simulink model "BMS"  (R2024b)
settings: Solver=ode23tb  StartTime=0.0  StopTime=1  RelTol=1e-3  EnableMultiTasking=on
PreLoadFcn:
  | % Data of Solar Panel
  | %5000[W]/130[W]
  | % Total power generated by solar panel reaches 5[KW].
  | % each solar panel generates power 130[kW].
  | V = [0    40 80 120 160 180 200 217 240 260 280];
  | I = 5000/130*[0.68 0.675 0.67 0.665 0.660 0.655 0.640 0.6 0.48 0.28 0];
  | 
  | %subplot(211);plot(V,I);xlabel('Voltage[V]');ylabel('Current[a]')
  | %subplot(212);plot(V.*I);title('Power[W]')
  | 
  | % Sample Time[s]
  | Ts =5e-6;
  | 
  | 
  | %MPPT + PV Control
  | % PI control pamameter of Voltage control(Outer loop)
  | Kp_V = 50e-3;
  | Ki_V = 10;
  | 
  | % PI Control pamameter of Current control(Inner loop)
  | Kp_I = 25e-3;
  | Ki_I = 10;
  | 
  | % Utility Interconnection Control
  | % PI Control pamameter of Voltage control(Outer loop)
  | Kp_V2 = 0.01;
  | Ki_V2 = 25;
  | 
  | % PI control pamameter of Current control(Inner loop)
  | Kp_I2 = 0.01;
  | Ki_I2 = 25;
  | 
  | 
  | % Difference of voltege using in MPPT
  | dV = 0.5;
  | 
  | % Battery Control
  | % PI Control pamameter of Voltage control(Outer loop)
  | Kp_VB = 0.4;
  | Ki_VB = 2;
  | 
  | % PI control pamameter of Current control(Inner loop)
  | Kp_IB = 0.1;
  | Ki_IB = 0.5;
undefined symbols (not defined in the file): Acid, Ion, Lead, Lithium, sigbuilder_block
libraries: spsBreakerLib x120, spsBatteryLib x111, spsSeriesRLCBranchLib x59, spsVoltageMeasurementLib x17, spsIdealSwitchLib x15, spsMosfetLib x11, slpidlib x9, spsCurrentMeasurementLib x7, spsPWMGeneratorDCDCLib x7, spsDiodeLib x6, spsPWMGenerator2LevelLib x5, spspowerguiLib x3
(part 1 of 6)
Description:
  | Copyright 2008-2017 The MathWorks, Inc.
settings Model: SimulationMode=accelerator  Creator=MathWorks  LastModifiedBy=Jatay
settings SolverCC: ZeroCrossControl=DisableAll  ZeroCrossAlgorithm=Adaptive  AlgebraicLoopSolver=TrustRegion
settings DataIOCC: LimitDataPoints=on  SaveFormat=Array  SignalLoggingSaveFormat=ModelDataLogs  ReturnWorkspaceOutputs=off
settings OptimizationCC: ExpressionDepthLimit=2147483647  LifeSpan=inf
settings DebuggingCC: UnderspecifiedInitializationDetection=Classic  MergeDetectMultiDrivingBlocksExec=none  SolverPrmCheckMsg=warning  FcnCallInpInsideContextMsg=warning  UnconnectedInputMsg=warning  UnconnectedOutputMsg=warning  UnconnectedLineMsg=warning  AllowSymbolicDim=off  StateNameClashWarn=warning  SFUnexpectedBacktrackingDiag=warning  SFNoUnconditionalDefaultTransitionDiag=warning  SFExecutionAtInitializationDiag=none  ArithmeticOperatorsInVariantConditions=warning
settings HardwareCC: ProdBitPerPointer=32  ProdBitPerSizeT=32  ProdBitPerPtrDiffT=32  ProdLargestAtomicFloat=None  ProdIntDivRoundTo=Undefined  ProdEndianess=Unspecified  ProdWordSize=32  ProdHWDeviceType=32-bit Generic
settings ModelReferenceCC: EnableRefExpFcnMdlSchedulingChecks=on  PropagateSignalLabelsOutOfModel=off
settings SFSimCC: SimUseLocalCustomCode=off  SimParseCustomCode=off  CustomCodeUndefinedFunction=UseInterfaceOnly
settings RTWCC: RTWUseLocalCustomCode=off  GPUComputeCapability=3.5
settings CodeAppCC: StateflowObjectComments=on
settings GRTTargetCC: TargetLangStandard=C89/C90 (ANSI)  CombineOutputUpdateFcns=off  GRTInterface=on
settings ConfigComp: CovMetricSettings=dw  CovSaveCumulativeToWorkspaceVar=on  CovSaveSingleToWorkspaceVar=on  CovExternalEMLEnable=off  CovSFcnEnable=off
settings SimscapeCC: SimscapeNormalizeSystem=off

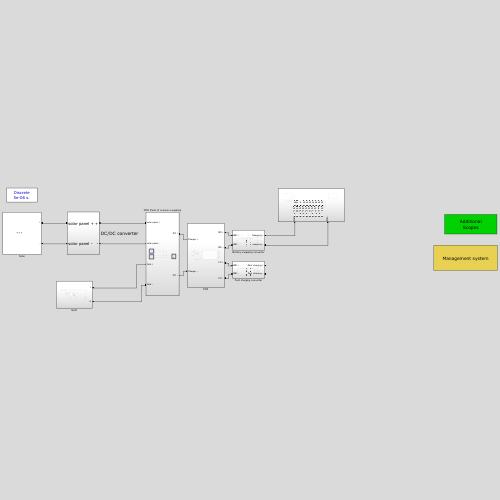
[thumbnail: Simulink's stored preview of the top-level diagram]
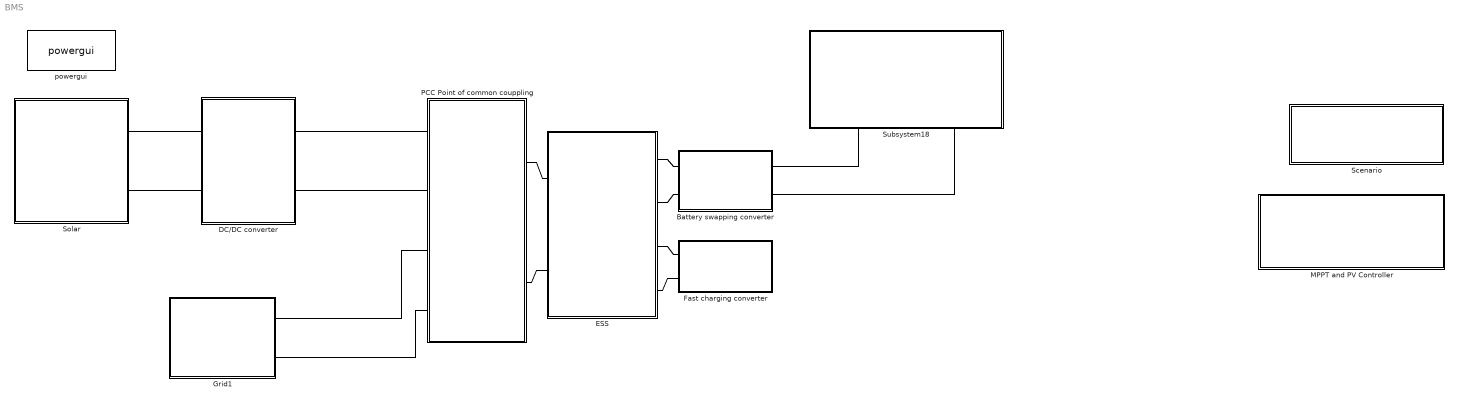
== system BMS ==
  Battery swapping converter : Subsystem
  DC/DC converter : Subsystem
  ESS : Subsystem
  Fast charging converter : Subsystem
  Grid1 : Subsystem
  MPPT and PV Controller : Subsystem
      mask Display: disp('Management system')
  PCC Point of common couppling : Subsystem
  Scenario : Subsystem
      mask Display: disp('Additional\nScopes')
  Solar : Subsystem
      mask Display: image('Solar-Power-Plant-1024x536.jpg');
  Subsystem18 : Subsystem
  powergui : spspowerguiLib/powergui  Priority=1  SimulationMode=Discrete  SampleTime=5e-6  frequency=60  Iterations=50  frequencyindice=0  Pbase=100e6  ErrMax=1e-4  UnitsV=kV  UnitsW=MW  buscounter=0  FunctionMessages=off  echomessages=off  EnableUseOfTLC=off  CurrentSourceSwitches=off  DisableSnubberDevices=off  DisableRonSwitches=off  DisableVfSwitches=off  DisplayEquations=off  AutomaticDiscreteSolvers=off  SolverType=Tustin  Interpol=off  ExternalGateDelay=off  methode=off  Ts=0  x0status=blocks  SPID=off  SwTol=0  HookPort=off  NonlinearTolerance=1e-4  nMaxIteration=100  ContinueOnMaxIteration=off  RestoreLinks=warning  ResistiveCurrentMeasurement=off  Frange=[0:2:500]  Ylog=off  Xlog=on  ShowGrid=off  save=off  variable=ZData  structure=0  ZoomFFT=off  StartTime=0.0  cycles=1  DisplayStyle=1  fundamental=60  FreqAxis=off  MaxFrequency=1000  frequencyindicesteady=1  RmsSteady=1  display=off
  connections:
  DC/DC converter/LConn2 -- Solar/RConn2
  DC/DC converter/LConn1 -- Solar/RConn1
  ESS/LConn2 -- PCC Point of common couppling/RConn2
  PCC Point of common couppling/RConn1 -- ESS/LConn1
  PCC Point of common couppling/LConn1 -- DC/DC converter/RConn1
  DC/DC converter/RConn2 -- PCC Point of common couppling/LConn2
  Grid1/RConn1 -- PCC Point of common couppling/LConn3
  Grid1/RConn2 -- PCC Point of common couppling/LConn4
  ESS/RConn1 -- Battery swapping converter/LConn1
  ESS/RConn2 -- Battery swapping converter/LConn2
  ESS/RConn3 -- Fast charging converter/LConn1
  Fast charging converter/LConn2 -- ESS/RConn4
  Subsystem18/LConn1 -- Battery swapping converter/RConn1
  Subsystem18/LConn2 -- Battery swapping converter/RConn2

== system BMS/Battery swapping converter ==
  Current Measurement : spsCurrentMeasurementLib/Current Measurement  PhasorSimulation=off  OutputType=Complex  PSBequivalent=0
  Current Measurement1 : spsCurrentMeasurementLib/Current Measurement  PhasorSimulation=off  OutputType=Complex  PSBequivalent=0
  Current Measurement2 : spsCurrentMeasurementLib/Current Measurement  PhasorSimulation=off  OutputType=Complex  PSBequivalent=0
  Diode : spsDiodeLib/Diode  Ron=0.001  Lon=0  Vf=0.8  IC=0  UseSnubber=0  Rs=500  Cs=250e-9  Measurements=off
  Mosfet : spsMosfetLib/Mosfet  Ron=0.1  Lon=0  Rd=0.01  Vfd=0  IC=0  Rs=1e5  Cs=inf  Measurements=off
  Product : Product
  Pulse Generator : DiscretePulseGenerator  PulseType=Time based  Period=10  PulseWidth=5
  Scope2 : Scope  NumInputPorts=3
  Scope3 : Scope
  Scope4 : Scope
  Series RLC Branch : spsSeriesRLCBranchLib/Series RLC Branch  LConnTagsString=__new0  RConnTagsString=__new0  BranchType=L  Resistance=1  Inductance=1e-3  SetiL0=off  InitialCurrent=0  Capacitance=1e-6  Setx0=off  InitialVoltage=0  Measurements=None
  Series RLC Branch2 : spsSeriesRLCBranchLib/Series RLC Branch  LConnTagsString=__new0  RConnTagsString=__new0  BranchType=C  Resistance=1  Inductance=1e-3  SetiL0=off  InitialCurrent=0  Capacitance=1e-6  Setx0=off  InitialVoltage=0  Measurements=None
  Voltage Measurement : spsVoltageMeasurementLib/Voltage Measurement  PhasorSimulation=off  OutputType=Complex  PSBequivalent=0
  BB + : PMIOPort  Side=Left
  BB - : PMIOPort  Port=2  Side=Left
  Swapping + : PMIOPort  Port=3  Side=Right
  swapping - : PMIOPort  Port=4  Side=Right
  wires:
  Current Measurement/1 -> Scope2/1
  Voltage Measurement/1 -> Scope4/1, Product/1
  Current Measurement1/1 -> Scope2/3, Product/2
  Product/1 -> Scope3/1
  Current Measurement2/1 -> Scope2/2
  Pulse Generator/1 -> Mosfet/1
  connections:
  Series RLC Branch2/RConn1 -- BB -/RConn1 -- Series RLC Branch/RConn1 -- swapping -/RConn1 -- Voltage Measurement/LConn2
  Diode/LConn1 -- Current Measurement1/LConn1 -- Series RLC Branch2/LConn1
  BB +/RConn1 -- Current Measurement/LConn1
  Current Measurement1/RConn1 -- Swapping +/RConn1 -- Voltage Measurement/LConn1
  Mosfet/RConn1 -- Diode/RConn1 -- Current Measurement2/LConn1
  Current Measurement/RConn1 -- Mosfet/LConn1
  Current Measurement2/RConn1 -- Series RLC Branch/LConn1

== system BMS/DC//DC converter ==
  Bidirectional DC/DC Converter : Subsystem
  DC - DC Converter : Subsystem
  DC bus : Subsystem
  Voltage Measurement2 : spsVoltageMeasurementLib/Voltage Measurement  PhasorSimulation=off  OutputType=Complex  PSBequivalent=0
  solar panel + : PMIOPort  Side=Left
  solar panel - : PMIOPort  Port=2  Side=Left
  + : PMIOPort  Port=3  Side=Right
  - : PMIOPort  Port=4  Side=Right
  tag scope: solar_controller=global
  wires:
  Voltage Measurement2/1 -> [solar_controller]
  connections:
  DC - DC Converter/RConn1 -- DC bus/LConn1
  solar panel +/RConn1 -- DC - DC Converter/LConn1 -- Voltage Measurement2/LConn1
  DC - DC Converter/LConn2 -- Voltage Measurement2/LConn2 -- solar panel -/RConn1
  DC - DC Converter/RConn2 -- DC bus/LConn2
  Bidirectional DC/DC Converter/LConn1 -- DC bus/RConn1
  Bidirectional DC/DC Converter/LConn2 -- DC bus/RConn2
  -/RConn1 -- Bidirectional DC/DC Converter/RConn2
  Bidirectional DC/DC Converter/RConn1 -- +/RConn1

== system BMS/ESS ==
  Display : Display
  Ideal Switch : spsIdealSwitchLib/Ideal Switch  Ron=0.001  Lon=0  IC=0  Rs=1e5  Cs=inf  Measurements=off
  Subsystem : Subsystem
  Charger + : PMIOPort  Side=Left
  Charger - : PMIOPort  Port=2  Side=Left
  BS + : PMIOPort  Port=3  Side=Right
  BS - : PMIOPort  Port=4  Side=Right
  FC + : PMIOPort  Port=5  Side=Right
  FC - : PMIOPort  Port=6  Side=Right
  wires:
  [ss] -> Display/1, Ideal Switch/1
  connections:
  Ideal Switch/LConn1 -- Charger +/RConn1
  Charger -/RConn1 -- Subsystem/LConn2
  Ideal Switch/RConn1 -- Subsystem/LConn1
  FC -/RConn1 -- BS -/RConn1 -- Subsystem/RConn2
  Subsystem/RConn1 -- BS +/RConn1 -- FC +/RConn1

== system BMS/Fast charging converter ==
  Current Measurement : spsCurrentMeasurementLib/Current Measurement  PhasorSimulation=off  OutputType=Complex  PSBequivalent=0
  Current Measurement1 : spsCurrentMeasurementLib/Current Measurement  PhasorSimulation=off  OutputType=Complex  PSBequivalent=0
  Current Measurement2 : spsCurrentMeasurementLib/Current Measurement  PhasorSimulation=off  OutputType=Complex  PSBequivalent=0
  Diode : spsDiodeLib/Diode  Ron=0.001  Lon=0  Vf=0.8  IC=0  UseSnubber=0  Rs=500  Cs=250e-9  Measurements=off
  Mosfet : spsMosfetLib/Mosfet  Ron=0.1  Lon=0  Rd=0.01  Vfd=0  IC=0  Rs=1e5  Cs=inf  Measurements=off
  Product : Product
  Pulse Generator : DiscretePulseGenerator  PulseType=Time based  Period=10  PulseWidth=5
  Scope2 : Scope  NumInputPorts=3
  Scope3 : Scope
  Scope4 : Scope
  Series RLC Branch : spsSeriesRLCBranchLib/Series RLC Branch  LConnTagsString=__new0  RConnTagsString=__new0  BranchType=L  Resistance=1  Inductance=1e-3  SetiL0=off  InitialCurrent=0  Capacitance=1e-6  Setx0=off  InitialVoltage=0  Measurements=None
  Series RLC Branch2 : spsSeriesRLCBranchLib/Series RLC Branch  LConnTagsString=__new0  RConnTagsString=__new0  BranchType=C  Resistance=1  Inductance=1e-3  SetiL0=off  InitialCurrent=0  Capacitance=1e-6  Setx0=off  InitialVoltage=0  Measurements=None
  Voltage Measurement : spsVoltageMeasurementLib/Voltage Measurement  PhasorSimulation=off  OutputType=Complex  PSBequivalent=0
  BB + : PMIOPort  Side=Left
  BB - : PMIOPort  Port=2  Side=Left
  Fast charging + : PMIOPort  Port=3  Side=Right
  Fast charging - : PMIOPort  Port=4  Side=Right
  wires:
  Current Measurement/1 -> Scope2/1
  Voltage Measurement/1 -> Scope4/1, Product/1
  Current Measurement1/1 -> Scope2/3, Product/2
  Product/1 -> Scope3/1
  Current Measurement2/1 -> Scope2/2
  Pulse Generator/1 -> Mosfet/1
  connections:
  Voltage Measurement/LConn2 -- Fast charging -/RConn1 -- Series RLC Branch2/RConn1 -- Series RLC Branch/RConn1 -- BB -/RConn1
  Diode/LConn1 -- Current Measurement1/LConn1 -- Series RLC Branch2/LConn1
  BB +/RConn1 -- Current Measurement/LConn1
  Current Measurement1/RConn1 -- Voltage Measurement/LConn1 -- Fast charging +/RConn1
  Mosfet/RConn1 -- Diode/RConn1 -- Current Measurement2/LConn1
  Current Measurement/RConn1 -- Mosfet/LConn1
  Current Measurement2/RConn1 -- Series RLC Branch/LConn1

== system BMS/Grid1 ==
  Display : Display
  Grid : spsThreePhaseSourceLib/Three-Phase Source  InternalConnection=Yg  VoltagePhases=off  Voltage=380  PhaseAngle=0  Voltage_phases=[25e3 25e3 25e3]/sqrt(3)  PhaseAngles_phases=[0 -120 +120]  Frequency=50  NonIdealSource=on  SpecifyImpedance=on  Resistance=0.8929  Inductance=16.58e-3  ShortCircuitLevel=100e6  BaseVoltage=380  XRratio=7  BusType=swing  Pref=10e3  Qref=0  Prefabc=[10e3, 10e3, 10e3]  Qrefabc=[0, 0, 0]  Qmin=-inf  Qmax=inf
  LOAD1 : spsThreePhaseSeriesRLCLoadLib/Three-Phase Series RLC Load  LConnTagsString=A|B|C  Configuration=Y (grounded)  NominalVoltage=380  Vabc=[1e3 1e3 1e3]  Vabcp=[1e3 1e3 1e3]  NominalFrequency=50  UnbalancedPower=off  ActivePower=1e3  InductivePower=0  CapacitivePower=0  Pabc=[10e3 9e3 11e3]  QLabc=[100 90 110]  QCabc=[100 90 110]  Pabcp=[10e3 9e3 11e3]  QLabcp=[100 90 110]  QCabcp=[100 90 110]  Measurements=None  LoadType=constant Z
  Measurement : spsThreePhaseVIMeasurementLib/Three-Phase V-I Measurement  VoltageMeasurement=phase-to-phase  SetLabelV=on  LabelV=Vabc_grid  Vpu=off  VpuLL=off  CurrentMeasurement=yes  SetLabelI=on  LabelI=Iabc_grid  Ipu=off  Pbase=100e6  Vbase=500e3  OutputType=Complex  PhasorSimulation=off  PSBequivalent=0
  Mux : Mux  Inputs=2
  Repeating Sequence Stair : simulink/Sources/Repeating Sequence Stair  OutValues=[0 0 1 1 0].'  tsamp=0.1  OutMin=[]  OutMax=[]  OutDataTypeStr=double  OutputDataTypeScalingMode=double  OutDataType=fixdt(0,8)  ConRadixGroup=Best Precision: Vector-wise  OutScaling=2^-12
  Scope : Scope
  Scope1 : Scope
  Scope2 : Scope  NumInputPorts=2
  V2G & G2V results : Scope  NumInputPorts=3
  Voltage Measurement : spsVoltageMeasurementLib/Voltage Measurement  PhasorSimulation=off  OutputType=Complex  PSBequivalent=0
  Wall charger Connection Box : Subsystem
  + : PMIOPort  Side=Right
  +1 : PMIOPort  Port=2  Side=Right
  tag scope: Control=global
  wires:
  [Control] -> Wall charger Connection Box/1(Control)
  Mux/1 -> V2G & G2V results/3
  [Vabc_grid] -> V2G & G2V results/1
  [Vabc_inv] -> V2G & G2V results/2
  Repeating Sequence Stair/1 -> [Control], Scope1/1
  [Vabc_inv] -> Mux/2
  [Iabc_out] -> Scope2/2
  [Iabc_inv] -> Scope/1
  [Vabc_out] -> Scope2/1
  Voltage Measurement/1 -> Display/1
  [Vabc_grid] -> Mux/1
  connections:
  Wall charger Connection Box/RConn2 -- Voltage Measurement/LConn2 -- +1/RConn1
  Grid/RConn1 -- Measurement/LConn1
  Grid/RConn3 -- Measurement/LConn3
  Wall charger Connection Box/RConn1 -- Voltage Measurement/LConn1 -- +/RConn1
  Grid/RConn2 -- Measurement/LConn2
  LOAD1/LConn3 -- Wall charger Connection Box/LConn3 -- Measurement/RConn3
  Measurement/RConn2 -- Wall charger Connection Box/LConn2 -- LOAD1/LConn2
  Measurement/RConn1 -- Wall charger Connection Box/LConn1 -- LOAD1/LConn1

== system BMS/MPPT and PV Controller ==
  Battery controller : Subsystem
  Inverter controller : Subsystem
  MMPT Controller : Subsystem
  Solar controller : Subsystem
  Swapping battery controller : Subsystem

== system BMS/PCC Point of common couppling ==
  note: ESS
  note: Grid
  note: Solar
  DC + : PMIOPort  Side=Right
  solar panel + : PMIOPort  Port=2  Side=Left
  solar panel - : PMIOPort  Port=3  Side=Left
  DC - : PMIOPort  Port=4  Side=Right
  Grid + : PMIOPort  Port=5  Side=Left
  Grid - : PMIOPort  Port=6  Side=Left
  connections:
  DC +/RConn1 -- solar panel +/RConn1 -- Grid +/RConn1
  solar panel -/RConn1 -- Grid -/RConn1 -- DC -/RConn1

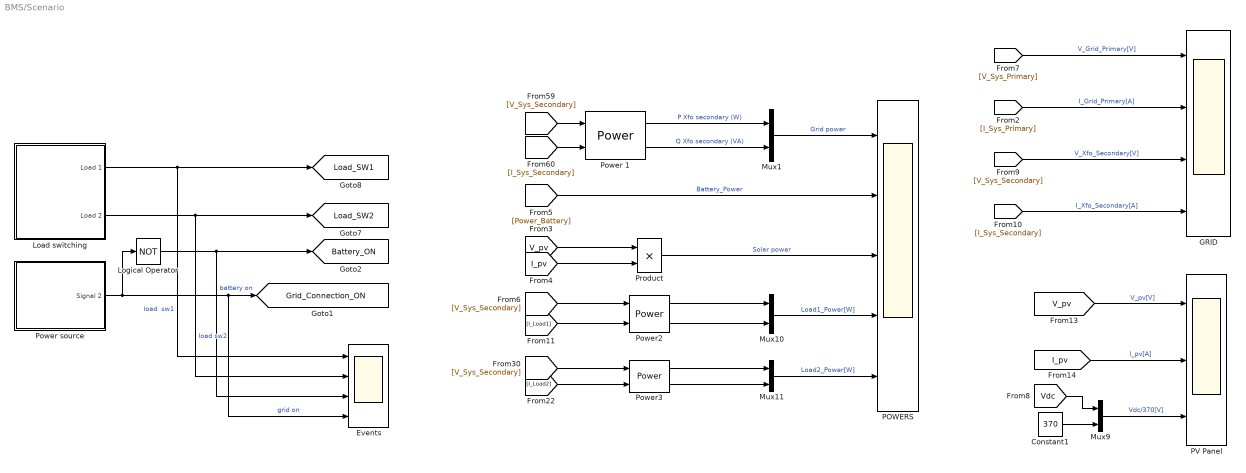
== system BMS/Scenario ==
  Constant1 : Constant  Value=370
  Events : Scope  NumInputPorts=4
  GRID : Scope  NumInputPorts=4
  Load switching : Subsystem  Tag=STV Subsys  LoadFcn=sigbuilder_block('load');  StartFcn=sigbuilder_block('start');  StopFcn=sigbuilder_block('stop');  ClipboardFcn=sigbuilder_block('clipboard');  mask(Sigbuilder block){tuvar=[0:10]}
      mask help: Simulink:masks:SigbuilderBlock_MD
      mask init:
      | if ~strcmp(get_param(bdroot(gcbh),'SimulationStatus'),'stopped') tuvar = sigbuilder_block('maskInit'); end
      settings: CopyFcn=sigbuilder_block('copy');  DeleteFcn=sigbuilder_block('delete');  ModelCloseFcn=sigbuilder_block('modelClose');  PreSaveFcn=sigbuilder_block('preSave');  PauseFcn=sigbuilder_block('pause');  ContinueFcn=sigbuilder_block('continue');  NameChangeFcn=sigbuilder_block('namechange');  OpenFcn=sigbuilder_block('open',[57 105.75 1180.5 663.75 ]);  CloseFcn=sigbuilder_block('close');
      mask Display: plot(0, 0, 100, 100,[2, 2, 32, 32, 2], [68, 8, 8, 68, 68],[32, 2], [38, 38], [32, 19, 2],[53, 60, 44], [32, 17, 17, 2],[16, 16, 31, 31]);txt = getActiveGroup(gcbh);text(2, 100, txt,'verticalAlignment', 'top');
  Logical Operator : Logic  Operator=NOT  AllPortsSameDT=off  OutDataTypeStr=boolean
  Mux{1,9..11} (4 alike) : Mux  Inputs=2
  POWERS : Scope  NumInputPorts=5
  PV Panel : Scope  NumInputPorts=3
  Power 1 : spsPowerLib/Power  Freq=60  Vinit=[1, 0]  Iinit=[1, 0]  Ts=0
  Power source : Subsystem  Tag=STV Subsys  LoadFcn=sigbuilder_block('load');  StartFcn=sigbuilder_block('start');  StopFcn=sigbuilder_block('stop');  ClipboardFcn=sigbuilder_block('clipboard');  mask(Sigbuilder block){tuvar=[0:10]}
      mask help: Simulink:masks:SigbuilderBlock_MD
      mask init:
      | if ~strcmp(get_param(bdroot(gcbh),'SimulationStatus'),'stopped') tuvar = sigbuilder_block('maskInit'); end
      settings: CopyFcn=sigbuilder_block('copy');  DeleteFcn=sigbuilder_block('delete');  ModelCloseFcn=sigbuilder_block('modelClose');  PreSaveFcn=sigbuilder_block('preSave');  PauseFcn=sigbuilder_block('pause');  ContinueFcn=sigbuilder_block('continue');  NameChangeFcn=sigbuilder_block('namechange');  OpenFcn=sigbuilder_block('open',[436.966 199.241 549.931 400.345 ]);  CloseFcn=sigbuilder_block('close');
      mask Display: plot(0, 0, 100, 100,[2, 2, 32, 32, 2], [68, 8, 8, 68, 68],[32, 2], [38, 38], [32, 19, 2],[53, 60, 44], [32, 17, 17, 2],[16, 16, 31, 31]);txt = getActiveGroup(gcbh);text(2, 100, txt,'verticalAlignment', 'top');
  Power2 : spsPowerLib/Power  Freq=60  Vinit=[1, 0]  Iinit=[1, 0]  Ts=0
  Power3 : spsPowerLib/Power  Freq=60  Vinit=[1, 0]  Iinit=[1, 0]  Ts=0
  Product : Product  RndMeth=Zero
  tag scope: Battery_ON=global, Grid_Connection_ON=global, Load_SW1=global, Load_SW2=global
  wires:
  Load switching/2(Load 2) -> [Load_SW2], Events/2  "load sw2"
  Logical Operator/1 -> Events/3, [Battery_ON]  "battery on"
  Power source/1(Signal 2) -> Events/4, [Grid_Connection_ON], Logical Operator/1  "grid on"
  Load switching/1(Load 1) -> [Load_SW1], Events/1  "load  sw1"
  [Vdc] -> Mux9/1
  Constant1/1 -> Mux9/2
  Mux9/1 -> PV Panel/3  "Vdc/370[V]"
  [V_Sys_Primary] -> GRID/1  "V_Grid_Primary[V]"
  [I_Sys_Primary] -> GRID/2  "I_Grid_Primary[A]"
  [V_Sys_Secondary] -> GRID/3  "V_Xfo_Secondary[V]"
  [I_Sys_Secondary] -> GRID/4  "I_Xfo_Secondary[A]"
  [V_pv] -> PV Panel/1  "V_pv[V]"
  [I_pv] -> PV Panel/2  "I_pv[A]"
  [V_pv] -> Product/1
  [I_pv] -> Product/2
  Product/1 -> POWERS/3  "Solar power"
  [Power_Battery] -> POWERS/2  "Battery_Power"
  [V_Sys_Secondary] -> Power 1/1
  [I_Sys_Secondary] -> Power 1/2
  [V_Sys_Secondary] -> Power2/1
  [I_Load1] -> Power2/2
  Mux10/1 -> POWERS/4  "Load1_Power[W]"
  [V_Sys_Secondary] -> Power3/1
  [I_Load2] -> Power3/2
  Mux11/1 -> POWERS/5  "Load2_Power[W]"
  Power2/1 -> Mux10/1
  Power2/2 -> Mux10/2
  Power3/1 -> Mux11/1
  Power3/2 -> Mux11/2
  Mux1/1 -> POWERS/1  "Grid power"
  Power 1/1 -> Mux1/1  "P Xfo secondary (W)"
  Power 1/2 -> Mux1/2  "Q Xfo secondary (VA)"

== system BMS/Solar ==
  note: 30 KW PV MPPT System
  "      " : ManualSwitch  CurrentSetting=0
  "      1" : ManualSwitch  CurrentSetting=0
  30 kW PV Array : spsPVArrayLib/PV Array  Npar=15  Nser=10  PlotType=array @ 1000 W/m2 & specified temperatures  S_vec="[ 1000  500  100 ]"  Temp_C_vec="[ 45 25  ]"  ModuleName=User-defined  PlotWhenSelected=off  Pm=213.15  Ncell=60  Voc=48  Isc=7.84  Vm=29  Im=7.35  beta_Voc_pc=-0.36099  alpha_Isc_pc=0.102  beta_Voc=-0.17328  alpha_Isc=0.0079968  IL=8.2285  I0=2.9956e-10  nI=1.2955  Rsh=7353.5939  Rs=2.0228  RobustModel=off  RobustCellTemperature=25  BAL=on  Tc=1e-6  Tfilter=5e-5
  Constant : Constant  Value=1000
  Constant3 : Constant  Value=25
  Current Measurement1 : spsCurrentMeasurementLib/Current Measurement  PhasorSimulation=off  OutputType=Complex  PSBequivalent=0
  Demux : Demux  Outputs=5
  Digital Clock : DigitalClock  SampleTime=0.001
  Diode : spsDiodeLib/Diode  Ron=0.5  Lon=0  Vf=0.7  IC=0  UseSnubber=0  Rs=1e5  Cs=250e-9  Measurements=off
  Diode1 : spsDiodeLib/Diode  Ron=0.5  Lon=0  Vf=0.7  IC=0  UseSnubber=0  Rs=1e5  Cs=250e-9  Measurements=off
  "Irradiance " : Subsystem  Tag=STV Subsys  LoadFcn=sigbuilder_block('load');  StartFcn=sigbuilder_block('start');  StopFcn=sigbuilder_block('stop');  ClipboardFcn=sigbuilder_block('clipboard');  mask(Sigbuilder block){tuvar=[0:10]}
      mask help: Sigbuilder GUI
      mask init:
      | if ~strcmp(get_param(bdroot(gcbh),'SimulationStatus'),'stopped') tuvar = sigbuilder_block('maskInit'); end
      settings: CopyFcn=sigbuilder_block('copy');  DeleteFcn=sigbuilder_block('delete');  ModelCloseFcn=sigbuilder_block('modelClose');  PreSaveFcn=sigbuilder_block('preSave');  PauseFcn=sigbuilder_block('pause')  ContinueFcn=sigbuilder_block('continue')  NameChangeFcn=sigbuilder_block('namechange');  OpenFcn=sigbuilder_block('open',[5.4 30 1141.2 507.6 ]);  CloseFcn=sigbuilder_block('close');
      mask Display: plot(0, 0, 100, 100,[2, 2, 32, 32, 2], [68, 8, 8, 68, 68],[32, 2], [38, 38], [32, 19, 2],[53, 60, 44], [32, 17, 17, 2],[16, 16, 31, 31]);txt = getActiveGroup(gcbh);text(2, 100, txt,'verticalAlignment', 'top');
  MPPT : Subsystem
  MPPT Power : Product
  Mosfet : spsMosfetLib/Mosfet  Ron=0.1  Lon=0  Rd=0.01  Vfd=0.7  IC=0  Rs=1e5  Cs=inf  Measurements=off
  Mux1 : Mux  Inputs=2
  PV Power : Product
  PWM Generator (DC-DC) : spsPWMGeneratorDCDCLib/PWM Generator (DC-DC)  Fsw=1500  Ts=0
  Scope : Scope  NumInputPorts=5
  Scope{1..3,5} (4 alike) : Scope
  Scope6 : Scope  NumInputPorts=3
  Scope7 : Scope  NumInputPorts=3
  Series RLC Branch : spsSeriesRLCBranchLib/Series RLC Branch  LConnTagsString=__new0  RConnTagsString=__new0  BranchType=L  Resistance=0.001  Inductance=0.4e-1  SetiL0=off  InitialCurrent=0  Capacitance=1e-6  Setx0=off  InitialVoltage=0  Measurements=None
  Series RLC Branch1 : spsSeriesRLCBranchLib/Series RLC Branch  LConnTagsString=__new0  RConnTagsString=__new0  BranchType=R  Resistance=11  Inductance=0.1  SetiL0=off  InitialCurrent=0  Capacitance=100e-6  Setx0=off  InitialVoltage=0  Measurements=None
  Series RLC Branch2 : spsSeriesRLCBranchLib/Series RLC Branch  LConnTagsString=__new0  RConnTagsString=__new0  BranchType=C  Resistance=6  Inductance=0.1  SetiL0=off  InitialCurrent=0  Capacitance=700e-5  Setx0=off  InitialVoltage=0  Measurements=None
  Series RLC Branch3 : spsSeriesRLCBranchLib/Series RLC Branch  LConnTagsString=__new0  RConnTagsString=__new0  BranchType=C  Resistance=6  Inductance=0.1  SetiL0=off  InitialCurrent=0  Capacitance=1000e-5  Setx0=off  InitialVoltage=0  Measurements=None
  Voltage Measurement : spsVoltageMeasurementLib/Voltage Measurement  PhasorSimulation=off  OutputType=Complex  PSBequivalent=0
  Voltage Measurement1 : spsVoltageMeasurementLib/Voltage Measurement  PhasorSimulation=off  OutputType=Complex  PSBequivalent=0
  + : PMIOPort  Side=Right
  - : PMIOPort  Port=2  Side=Right
  tag scope: I_pv=global, V_pv=global
  wires:
  Voltage Measurement/1 -> MPPT Power/2, Mux1/2, Scope7/2  "DC -DC Boost Converter Voltage"
  PWM Generator (DC-DC)/1 -> Mosfet/1
  Demux/1 -> Scope7/1, PV Power/1, [V_pv], MPPT/1("V _ PV "), Scope/1  "PV Voltage"
  Mux1/1 -> Scope1/1
  MPPT Power/1 -> Scope6/2, Scope2/1  "PO"
  Demux/2 -> PV Power/2, [I_pv], MPPT/2(I_PV), Scope/2
  Current Measurement1/1 -> MPPT Power/1, Mux1/1
  Voltage Measurement1/1 -> Scope3/1
  Demux/3 -> Scope/3
  Demux/4 -> Scope6/3, Scope7/3, Scope/4  "Irradiance"
  Digital Clock/1 -> MPPT/3(clock)
  MPPT/1(Duty) -> PWM Generator (DC-DC)/1
  PV Power/1 -> Scope6/1, Scope5/1
  Demux/5 -> Scope/5
  "Irradiance "/2(Temp) -> "      1"/1
  Constant3/1 -> "      1"/2
  "Irradiance "/1(Ir) -> "      "/2
  Constant/1 -> "      "/1
  "      "/1 -> 30 kW PV Array/1
  "      1"/1 -> 30 kW PV Array/2
  30 kW PV Array/1 -> Demux/1
  connections:
  Voltage Measurement/LConn2 -- 30 kW PV Array/RConn2 -- Diode1/LConn1 -- Series RLC Branch2/RConn1 -- Mosfet/RConn1 -- Voltage Measurement1/LConn2 -- Series RLC Branch3/RConn1 -- Series RLC Branch1/RConn1 -- -/RConn1
  Current Measurement1/RConn1 -- Series RLC Branch1/LConn1 -- Voltage Measurement/LConn1 -- +/RConn1
  Diode/RConn1 -- Series RLC Branch3/LConn1 -- Current Measurement1/LConn1
  Voltage Measurement1/LConn1 -- Series RLC Branch/RConn1 -- Mosfet/LConn1 -- Diode/LConn1
  Series RLC Branch2/LConn1 -- 30 kW PV Array/RConn1 -- Diode1/RConn1 -- Series RLC Branch/LConn1

== system BMS/Subsystem18 ==
  note: B1
  note: B2
  note: B3
  note: B4
  note: B5
  note: B6
  note: B13
  note: B14
  note: B15
  note: B16
  note: B17
  note: B18
  note: B19
  note: B20
  note: B21
  note: B22
  note: B7
  note: B8
  note: B9
  note: B10
  note: B11
  note: B12
  note: B23
  note: B24
  note: B25
  note: B26
  note: B27
  note: B28
  note: B29
  note: B30
  . : Subsystem
  Display : Display
  Subsystem : Subsystem
  Subsystem10 : Subsystem
  Subsystem11 : Subsystem
  Subsystem12 : Subsystem
  Subsystem13 : Subsystem
  Subsystem14 : Subsystem
  Subsystem15 : Subsystem
  Subsystem16 : Subsystem
  Subsystem17 : Subsystem
  Subsystem18 : Subsystem
  Subsystem19 : Subsystem
  Subsystem2 : Subsystem
  Subsystem20 : Subsystem
  Subsystem21 : Subsystem
  Subsystem22 : Subsystem
  Subsystem23 : Subsystem
  Subsystem24 : Subsystem
  Subsystem25 : Subsystem
  Subsystem26 : Subsystem
  Subsystem27 : Subsystem
  Subsystem28 : Subsystem
  Subsystem29 : Subsystem
  Subsystem3 : Subsystem
  Subsystem4 : Subsystem
  Subsystem5 : Subsystem
  Subsystem6 : Subsystem
  Subsystem7 : Subsystem
  Subsystem8 : Subsystem
  Subsystem9 : Subsystem
  Swapping battery controller : Subsystem
  Voltage Measurement : spsVoltageMeasurementLib/Voltage Measurement  PhasorSimulation=off  OutputType=Complex  PSBequivalent=0
  powergui : spspowerguiLib/powergui  Priority=1  SimulationMode=Continuous  SampleTime=50e-6  frequency=60  Iterations=50  frequencyindice=0  Pbase=100e6  ErrMax=1e-4  UnitsV=kV  UnitsW=MW  buscounter=0  FunctionMessages=off  echomessages=off  EnableUseOfTLC=off  CurrentSourceSwitches=off  DisableSnubberDevices=off  DisableRonSwitches=off  DisableVfSwitches=off  DisplayEquations=off  AutomaticDiscreteSolvers=off  SolverType=Tustin/Backward Euler (TBE)  Interpol=off  ExternalGateDelay=off  methode=off  Ts=100  x0status=blocks  SPID=on  SwTol=0  HookPort=off  NonlinearTolerance=1e-4  nMaxIteration=100  ContinueOnMaxIteration=off  RestoreLinks=warning  ResistiveCurrentMeasurement=off  Frange=[0:2:500]  Ylog=off  Xlog=on  ShowGrid=off  save=off  variable=ZData  structure=0  ZoomFFT=off  StartTime=0.0  cycles=1  DisplayStyle=1  fundamental=60  FreqAxis=off  MaxFrequency=1000  frequencyindicesteady=1  RmsSteady=1  display=off
  BB + : PMIOPort  Side=Left
  BB - : PMIOPort  Port=2  Side=Left
  wires:
  Voltage Measurement/1 -> Display/1
  connections:
  ./RConn2 -- Subsystem21/RConn2 -- Subsystem19/RConn2 -- Subsystem9/RConn2 -- Subsystem8/RConn2 -- Subsystem11/RConn2 -- Subsystem12/RConn2 -- Subsystem10/RConn2 -- Subsystem6/RConn2 -- Subsystem13/RConn2 -- Subsystem14/RConn2 -- Subsystem7/RConn2 -- Subsystem17/RConn2 -- Subsystem28/RConn2 -- Subsystem27/RConn2 -- Subsystem16/RConn2 -- Subsystem26/RConn2 -- Subsystem23/RConn2 -- Subsystem22/RConn2 -- Subsystem25/RConn2 -- Subsystem24/RConn2 -- Subsystem18/RConn2 -- Subsystem20/RConn2 -- Subsystem2/RConn2 -- Subsystem/RConn2 -- Subsystem3/RConn2 -- Subsystem4/RConn2 -- Voltage Measurement/LConn2 -- BB -/RConn1
  Subsystem10/RConn1 -- Subsystem7/RConn1 -- Subsystem17/RConn1 -- Subsystem29/RConn1 -- Subsystem29/RConn2 -- Subsystem28/RConn1 -- Subsystem27/RConn1 -- Subsystem16/RConn1 -- Subsystem26/RConn1 -- Subsystem25/RConn1 -- Subsystem22/RConn1 -- Subsystem23/RConn1 -- Subsystem24/RConn1 -- Subsystem15/RConn1 -- Subsystem15/RConn2 -- Subsystem14/RConn1 -- Subsystem13/RConn1 -- Subsystem6/RConn1 -- Subsystem12/RConn1 -- Subsystem11/RConn1 -- Subsystem8/RConn1 -- Subsystem20/RConn1 -- Voltage Measurement/LConn1 -- BB +/RConn1 -- ./RConn1 -- Subsystem5/RConn1 -- Subsystem5/RConn2 -- Subsystem4/RConn1 -- Subsystem3/RConn1 -- Subsystem/RConn1 -- Subsystem2/RConn1 -- Subsystem21/RConn1 -- Subsystem18/RConn1 -- Subsystem19/RConn1 -- Subsystem9/RConn1

== system BMS/DC//DC converter/Bidirectional DC//DC Converter ==
  C : spsSeriesRLCBranchLib/Series RLC Branch  LConnTagsString=__new0  RConnTagsString=__new0  BranchType=C  Resistance=1  Inductance=1e-3  SetiL0=off  InitialCurrent=0  Capacitance=1000e-6  Setx0=on  InitialVoltage=200  Measurements=None
  IGBT1 : spsIGBTDiodeLib/IGBT//Diode  Ron=1e-3  Rs=1e5  Cs=inf  Measurements=off
  IGBT2 : spsIGBTDiodeLib/IGBT//Diode  Ron=1e-3  Rs=1e5  Cs=inf  Measurements=off
  L : spsSeriesRLCBranchLib/Series RLC Branch  LConnTagsString=__new0  RConnTagsString=__new0  BranchType=L  Resistance=1  Inductance=470e-6*5  SetiL0=off  InitialCurrent=0  Capacitance=1000e-6  Setx0=off  InitialVoltage=0  Measurements=None
  Switch{1..4} (4 alike) : spsIdealSwitchLib/Ideal Switch  Ron=0.001  Lon=0  IC=0  Rs=1e6  Cs=inf  Measurements=off
  Batt + : PMIOPort  Side=Left
  Batt - : PMIOPort  Port=2  Side=Left
  + : PMIOPort  Port=3  Side=Right
  - : PMIOPort  Port=4  Side=Right
  wires:
  [G2_B] -> IGBT2/1
  [G1_B] -> IGBT1/1
  [Battery_ON] -> Switch3/1
  [Battery_ON] -> Switch1/1, Switch2/1
  [Battery_ON] -> Switch4/1
  connections:
  IGBT2/LConn1 -- L/RConn1 -- IGBT1/RConn1
  L/LConn1 -- Switch3/LConn1 -- C/LConn1
  Switch3/RConn1 -- +/RConn1
  Switch4/RConn1 -- -/RConn1
  Switch1/RConn1 -- IGBT1/LConn1
  Switch4/LConn1 -- C/RConn1 -- IGBT2/RConn1 -- Switch2/RConn1
  Batt -/RConn1 -- Switch2/LConn1
  Switch1/LConn1 -- Batt +/RConn1

== system BMS/DC//DC converter/DC - DC Converter ==
  C : spsSeriesRLCBranchLib/Series RLC Branch  LConnTagsString=__new0  RConnTagsString=__new0  BranchType=C  Resistance=0.01  Inductance=1e-3  SetiL0=off  InitialCurrent=0  Capacitance=1000e-6  Setx0=on  InitialVoltage=200  Measurements=None
  Diode : spsDiodeLib/Diode  Ron=0.001  Lon=0  Vf=1.1  IC=0  UseSnubber=off  Rs=500  Cs=250e-9  Measurements=off
  Diode2 : spsDiodeLib/Diode  Ron=0.001  Lon=0  Vf=0.7  IC=0  UseSnubber=off  Rs=500  Cs=250e-9  Measurements=off
  IGBT : spsIGBTLib/IGBT  Ron=0.001  Lon=0  Vf=1.1  Tf=1e-6  Tt=2e-6  IC=0  Rs=1e5  Cs=inf  Measurements=off
  RL : spsSeriesRLCBranchLib/Series RLC Branch  LConnTagsString=__new0  RConnTagsString=__new0  BranchType=RL  Resistance=0.05  Inductance=470e-6  SetiL0=off  InitialCurrent=0  Capacitance=1e-6  Setx0=off  InitialVoltage=0  Measurements=None
  DC + : PMIOPort  Side=Right
  solar panel + : PMIOPort  Port=2  Side=Left
  solar panel - : PMIOPort  Port=3  Side=Left
  DC - : PMIOPort  Port=4  Side=Right
  wires:
  [Pulse_PV] -> IGBT/1
  connections:
  Diode/RConn1 -- DC +/RConn1
  Diode2/RConn1 -- C/LConn1 -- RL/LConn1
  Diode/LConn1 -- RL/RConn1 -- IGBT/LConn1
  solar panel +/RConn1 -- Diode2/LConn1
  C/RConn1 -- solar panel -/RConn1 -- DC -/RConn1 -- IGBT/RConn1

== system BMS/DC//DC converter/DC bus ==
  1 ohm 2000uH : spsSeriesRLCBranchLib/Series RLC Branch  LConnTagsString=__new0  RConnTagsString=__new0  BranchType=RC  Resistance=1  Inductance=0  SetiL0=off  InitialCurrent=0  Capacitance=2000e-6  Setx0=on  InitialVoltage=370  Measurements=None
  RL + : spsSeriesRLCBranchLib/Series RLC Branch  LConnTagsString=__new0  RConnTagsString=__new0  BranchType=RL  Resistance=0.05  Inductance=470e-6  SetiL0=off  InitialCurrent=0  Capacitance=1e-6  Setx0=off  InitialVoltage=0  Measurements=None
  RL - : spsSeriesRLCBranchLib/Series RLC Branch  LConnTagsString=__new0  RConnTagsString=__new0  BranchType=RL  Resistance=0.05  Inductance=470e-6  SetiL0=off  InitialCurrent=0  Capacitance=1e-6  Setx0=off  InitialVoltage=0  Measurements=None
  Transfer Fcn : TransferFcn  Denominator=[1e-4 1]
  V : spsVoltageMeasurementLib/Voltage Measurement  PhasorSimulation=off  OutputType=Complex  PSBequivalent=0
  left + : PMIOPort  Side=Left
  left - : PMIOPort  Port=2  Side=Left
  right + : PMIOPort  Port=3  Side=Right
  right - : PMIOPort  Port=4  Side=Right
  tag scope: Vdc=global
  wires:
  V/1 -> Transfer Fcn/1
  Transfer Fcn/1 -> [Vdc]
  connections:
  RL +/RConn1 -- 1 ohm 2000uH/LConn1 -- right +/RConn1 -- V/LConn1
  RL -/RConn1 -- 1 ohm 2000uH/RConn1 -- right -/RConn1 -- V/LConn2
  left +/RConn1 -- RL +/LConn1
  left -/RConn1 -- RL -/LConn1

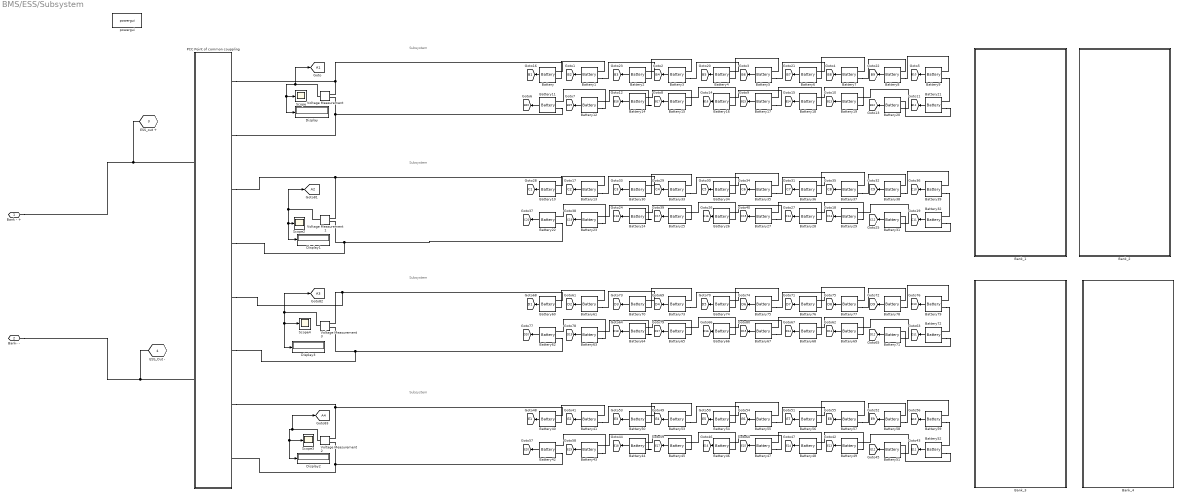
== system BMS/ESS/Subsystem ==
  note: Subsystem
  note: Subsystem
  note: Subsystem
  note: Subsystem
  Bank_1 : Subsystem
  Bank_2 : Subsystem
  Bank_3 : Subsystem
  Bank_4 : Subsystem
  Battery{,1..79} (80 alike) : spsBatteryLib/Battery  BatType=Lead-Acid  NomV=12  NomQ=100  SOC=80  Batt_Tr=10  PresetModel=on  MaxQ=104.1667  MinV=9  FullV=13.0658  Dis_rate=20  R=0.0012  Normal_OP=31.0278  expZone="[12.2171     0.333333]"
  Display{,1..3} (4 alike) : Display
  PCC Point of common couppling : Subsystem
  Scope{,2..4} (4 alike) : Scope
  Voltage Measurement{,1..3} (4 alike) : spsVoltageMeasurementLib/Voltage Measurement  PhasorSimulation=off  OutputType=Complex  PSBequivalent=0
  powergui : spspowerguiLib/powergui  Priority=1  SimulationMode=Continuous  SampleTime=50e-6  frequency=60  Iterations=50  frequencyindice=0  Pbase=100e6  ErrMax=1e-4  UnitsV=kV  UnitsW=MW  buscounter=0  FunctionMessages=off  echomessages=off  EnableUseOfTLC=off  CurrentSourceSwitches=off  DisableSnubberDevices=off  DisableRonSwitches=off  DisableVfSwitches=off  DisplayEquations=off  AutomaticDiscreteSolvers=off  SolverType=Tustin/Backward Euler (TBE)  Interpol=off  ExternalGateDelay=off  methode=off  Ts=100  x0status=blocks  SPID=on  SwTol=0  HookPort=off  NonlinearTolerance=1e-4  nMaxIteration=100  ContinueOnMaxIteration=off  RestoreLinks=warning  ResistiveCurrentMeasurement=off  Frange=[0:2:500]  Ylog=off  Xlog=on  ShowGrid=off  save=off  variable=ZData  structure=0  ZoomFFT=off  StartTime=0.0  cycles=1  DisplayStyle=1  fundamental=60  FreqAxis=off  MaxFrequency=1000  frequencyindicesteady=1  RmsSteady=1  display=off
  Bank - + : PMIOPort  Side=Left
  Bank- - : PMIOPort  Port=2  Side=Left
  ESS_out + : PMIOPort  Port=3  Side=Right
  ESS_Out - : PMIOPort  Port=4  Side=Right
  tag scope: A1=global, A2=global, A3=global, A4=global, B10=global, B11=global, B12=global, B13=global, B14=global, B15=global, B16=global, B17=global, B18=global, B19=global, B1=global, B20=global, B2=global, B3=global, B4=global, B5=global, B6=global, B7=global, B8=global, B9=global, C10=global, C11=global, C12=global, C13=global, C14=global, C15=global, C16=global, C17=global, C18=global, C19=global, C1=global, C20=global, C2=global, C3=global, C4=global, C5=global, C6=global, C7=global, C8=global, C9=global, D10=global, D11=global, D12=global, D13=global, D14=global, D15=global, D16=global, D17=global, D18=global, D19=global, D1=global, D20=global, D2=global, D3=global, D4=global, D5=global, D6=global, D7=global, D8=global, D9=global, E10=global, E11=global, E12=global, E13=global, E14=global, E15=global, E16=global, E17=global, E18=global, E19=global, E1=global, E20=global, E2=global, E3=global, E4=global, E5=global, E6=global, E7=global, E8=global, E9=global
  wires:
  Voltage Measurement/1 -> [A1], Scope/1, Display/1
  Battery1/1 -> [B2]
  Battery5/1 -> [B6]
  Battery25/1 -> [C17]
  Battery53/1 -> [E4]
  Battery20/1 -> [B12]
  Battery34/1 -> [C5]
  Battery28/1 -> [C14]
  Battery4/1 -> [B5]
  Battery45/1 -> [E17]
  Battery56/1 -> [E7]
  Voltage Measurement2/1 -> [A4], Scope3/1, Display2/1
  Battery16/1 -> [B16]
  Battery2/1 -> [B3]
  Battery18/1 -> [B14]
  Battery14/1 -> [B18]
  Voltage Measurement3/1 -> [A3], Display3/1, Scope4/1
  Battery8/1 -> [B9]
  Battery6/1 -> [B7]
  Battery17/1 -> [B15]
  Battery79/1 -> [D10]
  Battery65/1 -> [D17]
  Battery24/1 -> [C18]
  Battery9/1 -> [B10]
  Battery12/1 -> [B19]
  Battery61/1 -> [D2]
  Battery15/1 -> [B17]
  Battery21/1 -> [B11]
  Battery57/1 -> [E8]
  Battery11/1 -> [B20]
  Battery10/1 -> [C1]
  Battery64/1 -> [D18]
  Battery19/1 -> [B13]
  Battery73/1 -> [D4]
  Battery3/1 -> [B4]
  Battery41/1 -> [E2]
  Battery7/1 -> [B8]
  Battery49/1 -> [E13]
  Battery55/1 -> [E6]
  Battery66/1 -> [D16]
  Battery44/1 -> [E18]
  Battery58/1 -> [E9]
  Battery74/1 -> [D5]
  Battery42/1 -> [E20]
  Battery27/1 -> [C15]
  Battery43/1 -> [E19]
  Battery54/1 -> [E5]
  Battery48/1 -> [E14]
  Battery47/1 -> [E15]
  Battery13/1 -> [C2]
  Battery52/1 -> [E11]
  Battery59/1 -> [E10]
  Battery51/1 -> [E12]
  Battery/1 -> [B1]
  Battery50/1 -> [E3]
  Battery40/1 -> [E1]
  Battery46/1 -> [E16]
  Voltage Measurement1/1 -> [A2], Display1/1, Scope2/1
  Battery63/1 -> [D19]
  Battery38/1 -> [C9]
  Battery22/1 -> [C20]
  Battery39/1 -> [C10]
  Battery71/1 -> [D12]
  Battery32/1 -> [C11]
  Battery37/1 -> [C8]
  Battery33/1 -> [C4]
  Battery60/1 -> [D1]
  Battery35/1 -> [C6]
  Battery23/1 -> [C19]
  Battery29/1 -> [C13]
  Battery69/1 -> [D13]
  Battery31/1 -> [C12]
  Battery36/1 -> [C7]
  Battery30/1 -> [C3]
  Battery26/1 -> [C16]
  Battery70/1 -> [D3]
  Battery68/1 -> [D14]
  Battery75/1 -> [D6]
  Battery72/1 -> [D11]
  Battery62/1 -> [D20]
  Battery77/1 -> [D8]
  Battery67/1 -> [D15]
  Battery76/1 -> [D7]
  Battery78/1 -> [D9]
  connections:
  Battery61/LConn2 -- Battery70/LConn1
  Battery7/LConn2 -- Battery8/LConn1
  Battery54/LConn2 -- Battery55/LConn1
  Battery63/LConn2 -- Battery62/LConn1
  Voltage Measurement3/LConn2 -- Battery62/LConn2 -- PCC Point of common couppling/LConn6
  Battery20/LConn2 -- Battery19/LConn1
  Battery9/LConn2 -- Battery21/LConn1
  Battery56/LConn2 -- Battery57/LConn1
  Battery43/LConn2 -- Battery42/LConn1
  Battery/LConn1 -- PCC Point of common couppling/LConn1 -- Voltage Measurement/LConn1
  Battery40/LConn1 -- Voltage Measurement2/LConn1 -- PCC Point of common couppling/LConn7
  PCC Point of common couppling/LConn2 -- Battery11/LConn2 -- Voltage Measurement/LConn2
  Voltage Measurement3/LConn1 -- Battery60/LConn1 -- PCC Point of common couppling/LConn5
  Battery68/LConn2 -- Battery67/LConn1
  Battery2/LConn2 -- Battery3/LConn1
  Battery13/LConn2 -- Battery30/LConn1
  Battery39/LConn2 -- Battery32/LConn1
  Battery15/LConn2 -- Battery14/LConn1
  Battery16/LConn2 -- Battery15/LConn1
  Battery42/LConn2 -- Voltage Measurement2/LConn2 -- PCC Point of common couppling/LConn8
  Battery52/LConn2 -- Battery51/LConn1
  Battery14/LConn2 -- Battery12/LConn1
  Battery21/LConn2 -- Battery20/LConn1
  Battery6/LConn2 -- Battery7/LConn1
  Battery12/LConn2 -- Battery11/LConn1
  Battery18/LConn2 -- Battery17/LConn1
  Battery17/LConn2 -- Battery16/LConn1
  Battery3/LConn2 -- Battery4/LConn1
  Battery19/LConn2 -- Battery18/LConn1
  Battery53/LConn2 -- Battery54/LConn1
  Battery8/LConn2 -- Battery9/LConn1
  Battery26/LConn2 -- Battery25/LConn1
  Battery1/LConn2 -- Battery2/LConn1
  Battery60/LConn2 -- Battery61/LConn1
  Battery69/LConn2 -- Battery68/LConn1
  Battery50/LConn2 -- Battery53/LConn1
  Battery4/LConn2 -- Battery5/LConn1
  Battery5/LConn2 -- Battery6/LConn1
  Battery/LConn2 -- Battery1/LConn1
  Battery41/LConn2 -- Battery50/LConn1
  Battery49/LConn2 -- Battery48/LConn1
  Battery58/LConn2 -- Battery59/LConn1
  Battery48/LConn2 -- Battery47/LConn1
  Battery57/LConn2 -- Battery58/LConn1
  Battery55/LConn2 -- Battery56/LConn1
  Battery45/LConn2 -- Battery44/LConn1
  Battery40/LConn2 -- Battery41/LConn1
  Battery46/LConn2 -- Battery45/LConn1
  Battery59/LConn2 -- Battery52/LConn1
  Battery44/LConn2 -- Battery43/LConn1
  Battery76/LConn2 -- Battery77/LConn1
  Battery51/LConn2 -- Battery49/LConn1
  Battery47/LConn2 -- Battery46/LConn1
  Battery23/LConn2 -- Battery22/LConn1
  Battery10/LConn1 -- Voltage Measurement1/LConn1 -- PCC Point of common couppling/LConn3
  Battery25/LConn2 -- Battery24/LConn1
  Battery70/LConn2 -- Battery73/LConn1
  Battery10/LConn2 -- Battery13/LConn1
  Battery72/LConn2 -- Battery71/LConn1
  Battery28/LConn2 -- Battery27/LConn1
  Battery73/LConn2 -- Battery74/LConn1
  Battery74/LConn2 -- Battery75/LConn1
  Battery29/LConn2 -- Battery28/LConn1
  Battery33/LConn2 -- Battery34/LConn1
  Battery32/LConn2 -- Battery31/LConn1
  Voltage Measurement1/LConn2 -- Battery22/LConn2 -- PCC Point of common couppling/LConn4
  Battery30/LConn2 -- Battery33/LConn1
  Battery34/LConn2 -- Battery35/LConn1
  Battery38/LConn2 -- Battery39/LConn1
  Battery35/LConn2 -- Battery36/LConn1
  Battery24/LConn2 -- Battery23/LConn1
  Battery31/LConn2 -- Battery29/LConn1
  Battery36/LConn2 -- Battery37/LConn1
  Battery66/LConn2 -- Battery65/LConn1
  Battery37/LConn2 -- Battery38/LConn1
  Battery79/LConn2 -- Battery72/LConn1
  Battery27/LConn2 -- Battery26/LConn1
  Battery67/LConn2 -- Battery66/LConn1
  Battery77/LConn2 -- Battery78/LConn1
  Battery65/LConn2 -- Battery64/LConn1
  Battery78/LConn2 -- Battery79/LConn1
  Battery71/LConn2 -- Battery69/LConn1
  Battery64/LConn2 -- Battery63/LConn1
  Battery75/LConn2 -- Battery76/LConn1
  Bank - +/RConn1 -- ESS_out +/RConn1 -- PCC Point of common couppling/RConn1
  Bank- -/RConn1 -- ESS_Out -/RConn1 -- PCC Point of common couppling/RConn2

== system BMS/Grid1/Wall charger Connection Box ==
  Control : Inport
  Battery Switching Control : Subsystem
      settings: PortSchema="{\"entries\":[{\"content\":{\"sides\":[{\"content\":{\"connectorIds\":[\"LConn1\",\"LConn2\",\"LConn3\",\"LConn4\"]},\"type\":\"ConnectorPlacement.EquallySpacedRectSide\",\"uuid\":\"597ce45f-d2da-489f-9702-c83ae9b1152a\"},{\"content\":{\"connectorIds\":[\"In1\",\"RConn1\",\"RConn2\"],\"side\":\"RIGHT\"},\"type\":\"ConnectorPlacement.EquallySpacedRectSide\",\"uuid\":\"90ab1945-2787-45d6-b647-1c8eb49fe34d\"},{\"content\":{\"connectorIds\":[],\"side\":\"TOP\"},\"type\":\"ConnectorPlacement.EquallySpacedRectSide\",\"uuid\":\"5514c8fd-a1bb-4ed7-b1c0-08bce6a0e9e5\"}]},\"type\":\"ConnectorPlacement.EquallySpacedConnector\",\"uuid\":\"b6d566cb-31ba-40ab-ae9a-003997b713cb\"}],\"packageUris\":[\"http://schema.mathworks.com/mf0/Connector/R2020b\"],\"version\":\"1.0\"}"
  Buck-Boost Converter : Subsystem
  Connection Control : Subsystem
      settings: PortSchema="{\"entries\":[{\"content\":{\"sides\":[{\"content\":{\"connectorIds\":[\"LConn1\",\"LConn2\",\"LConn3\"]},\"type\":\"ConnectorPlacement.EquallySpacedRectSide\",\"uuid\":\"27ebf5cb-61b2-431e-8de2-c9344a0dfca5\"},{\"content\":{\"connectorIds\":[\"In1\",\"RConn1\",\"RConn2\",\"RConn3\",\"RConn4\",\"RConn5\",\"RConn6\"],\"side\":\"RIGHT\"},\"type\":\"ConnectorPlacement.EquallySpacedRectSide\",\"uuid\":\"2438100a-e43b-42f7-afa1-1af449516139\"},{\"content\":{\"connectorIds\":[],\"side\":\"TOP\"},\"type\":\"ConnectorPlacement.EquallySpacedRectSide\",\"uuid\":\"dcfa608d-f6dc-42e3-abf8-45a08af22825\"}]},\"type\":\"ConnectorPlacement.EquallySpacedConnector\",\"uuid\":\"5f0f36e8-f735-4489-a6f2-39fec655b509\"}],\"packageUris\":[\"http://schema.mathworks.com/mf0/Connector/R2020b\"],\"version\":\"1.0\"}"
  DC-AC / AC-DC Converter : Subsystem
  DC-DC converter with battery controller : Subsystem
  Grid_R : PMIOPort  Side=Left
  Grid_Y : PMIOPort  Port=2  Side=Left
  Grid_B : PMIOPort  Port=3  Side=Left
  Vehicle+ : PMIOPort  Port=4  Side=Right
  Vehicle- : PMIOPort  Port=5  Side=Right
  wires:
  Control/1 -> Connection Control/1(Control), Battery Switching Control/1(Control)
  connections:
  DC-AC / AC-DC Converter/LConn5 -- Connection Control/RConn5
  DC-AC / AC-DC Converter/LConn2 -- Connection Control/RConn2
  DC-DC converter with battery controller/RConn3 -- Battery Switching Control/LConn3
  Buck-Boost Converter/RConn2 -- DC-DC converter with battery controller/LConn2
  Grid_B/RConn1 -- Connection Control/LConn3
  DC-AC / AC-DC Converter/RConn3 -- Buck-Boost Converter/LConn3
  Grid_R/RConn1 -- Connection Control/LConn1
  DC-AC / AC-DC Converter/LConn1 -- Connection Control/RConn1
  Vehicle-/RConn1 -- Battery Switching Control/RConn2
  Vehicle+/RConn1 -- Battery Switching Control/RConn1
  Buck-Boost Converter/RConn4 -- DC-DC converter with battery controller/LConn4
  Grid_Y/RConn1 -- Connection Control/LConn2
  DC-AC / AC-DC Converter/LConn4 -- Connection Control/RConn4
  DC-DC converter with battery controller/RConn2 -- Battery Switching Control/LConn2
  DC-DC converter with battery controller/RConn1 -- Battery Switching Control/LConn1
  DC-DC converter with battery controller/RConn4 -- Battery Switching Control/LConn4
  Buck-Boost Converter/RConn1 -- DC-DC converter with battery controller/LConn1
  Buck-Boost Converter/LConn2 -- DC-AC / AC-DC Converter/RConn2
  DC-AC / AC-DC Converter/LConn3 -- Connection Control/RConn3
  DC-AC / AC-DC Converter/RConn1 -- Buck-Boost Converter/LConn1
  DC-AC / AC-DC Converter/RConn4 -- Buck-Boost Converter/LConn4
  Buck-Boost Converter/RConn3 -- DC-DC converter with battery controller/LConn3
  Connection Control/RConn6 -- DC-AC / AC-DC Converter/LConn6

== system BMS/MPPT and PV Controller/Battery controller ==
  Battery Controller : Subsystem
  Constant3 : Constant  Value=370
  PWM Controller 2 : Subsystem
  Transfer Fcn : TransferFcn  Denominator=[1e-2 1]
  Transfer Fcn2 : TransferFcn  Denominator=[1e-5 1]
  Transfer Fcn3 : TransferFcn  Denominator=[0.01 1]
  tag scope: G1_B=global, G2_B=global, Pulse_B=global
  wires:
  Transfer Fcn2/1 -> Battery Controller/3(I_bt)
  Transfer Fcn/1 -> Battery Controller/1(V_Dc)
  [Battery_ON] -> PWM Controller 2/Enable
  [Vdc] -> Transfer Fcn3/1
  [Vdc] -> Transfer Fcn/1
  Constant3/1 -> Battery Controller/2(370)
  [Ibt] -> Transfer Fcn2/1
  PWM Controller 2/1(Pulse) -> [Pulse_B]
  Battery Controller/1(Pulse 1) -> [G2_B]
  Transfer Fcn3/1 -> PWM Controller 2/1(Vdc)
  Battery Controller/2(Pulse 2) -> [G1_B]

== system BMS/MPPT and PV Controller/Inverter controller ==
  Constant1 : Constant  Value=370
  Inverter Controller : Subsystem
  Transfer Fcn1 : TransferFcn  Denominator=[1e-5 1]
  Transfer Fcn8 : TransferFcn  Denominator=[1e-5 1]
  tag scope: Pulse_UI=global
  wires:
  Inverter Controller/1(Pulse) -> [Pulse_UI]
  Constant1/1 -> Inverter Controller/2(370)
  [I_Sys_Secondary] -> Transfer Fcn1/1
  Transfer Fcn1/1 -> Inverter Controller/4(I_Sys_Secondary)
  [Grid_Connection_ON] -> Inverter Controller/Enable
  [V_Sys_Secondary] -> Inverter Controller/3(V_Sys_Secondary)
  [Vdc] -> Transfer Fcn8/1
  Transfer Fcn8/1 -> Inverter Controller/1(V_Dc)

== system BMS/MPPT and PV Controller/MMPT Controller ==
  MPPT Controller : Stateflow chart  TreatAsAtomicUnit=on
  PV Controller : Subsystem
  Transfer Fcn5 : TransferFcn  Denominator=[1e-5 1]
  Transfer Fcn6 : TransferFcn  Denominator=[1e-5 1]
  tag scope: Pulse_PV=global
  wires:
  Transfer Fcn6/1 -> MPPT Controller/2(I_pv), PV Controller/2(I_pv)
  PV Controller/1(Pulse) -> [Pulse_PV]
  [V_pv] -> Transfer Fcn5/1
  Transfer Fcn5/1 -> MPPT Controller/1(V_pv), PV Controller/1(V_pv)
  [I_pv] -> Transfer Fcn6/1
  MPPT Controller/1(Vref) -> PV Controller/3(Vref)

== system BMS/MPPT and PV Controller/Solar controller ==
  Constant1 : Constant  Value=0
  Constant2 : Constant
  Display2 : Display
  Display3 : Display
  Switch : Switch  Threshold=150  SaturateOnIntegerOverflow=off  InputSameDT=off
  tag scope: ss=global
  wires:
  Constant2/1 -> Switch/1
  Switch/1 -> Display2/1, [ss]
  Constant1/1 -> Switch/3
  [solar_controller] -> Display3/1, Switch/2
